simulink model "FYP"  (R2023b)
settings: Solver=FixedStepAuto  StartTime=0.0  StopTime=Inf  RelTol=1e-3  EnableMultiTasking=on
libraries: canmsglib x26, raspberrypiCommlib x26
(part 2 of 4)

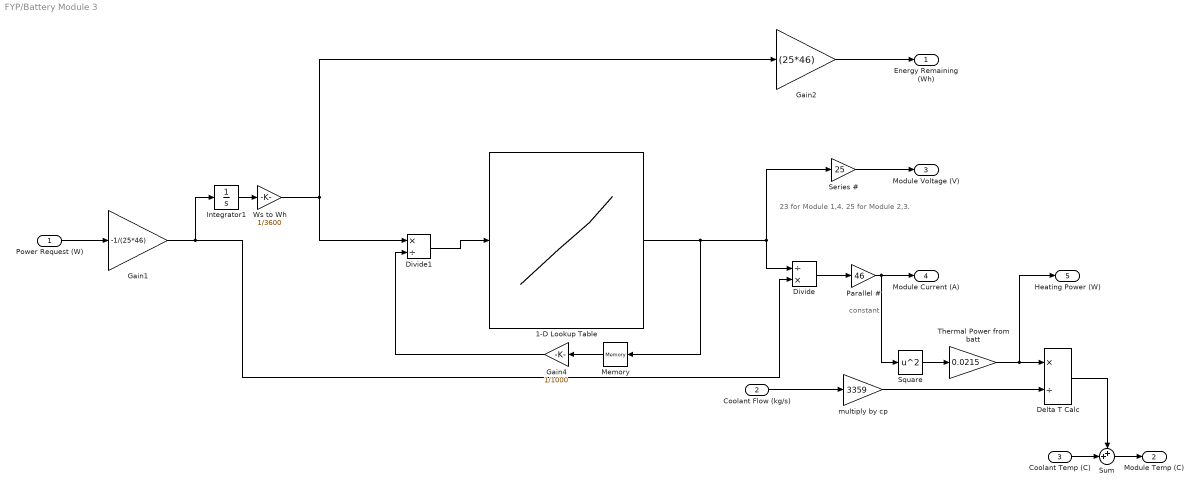
== system FYP/Battery Module 3 ==
  note: constant
  note: 23 for Module 1,4. 25 for Module 2,3.
  Power Request (W) : Inport
  Coolant Flow (kg/s) : Inport  Port=2
  Coolant Temp (C) : Inport  Port=3
  1-D Lookup Table : Lookup_n-D  NumberOfTableDimensions=1  BreakpointsForDimension1=|  Table=|  InternalRulePriority=Speed  RndMeth=Simplest
      BreakpointsForDimension1=|
      | [327.91963
      | 356.24194
      | 389.81097
      | 421.58966
      | 454.48731
      | 486.26599
      | 520.63596
      | 557.87992
      | 595.92482
      | 631.52398
      | 652.73854
      | 690.13124
      | 726.46639
      | 758.34729
      | 795.18499
      | 822.76755
      | 860.65393
      | 891.58806
      | 925.87788
      | 957.35139
      | 996.24173
      | 1029.9537
      | 1071.4861
      | 1113.3355
      | 1155.1849
      | 1197.0343
      | 1238.8837
      |  1280.733
      | 1322.5824
      | 1364.4318
      | 1406.2812
      | 1448.1306
      |   1489.98
      | 1531.8294
      | 1573.6788
      | 1615.5282
      | 1657.3776
      |  1699.227
      | 1741.0764
      | 1782.9257
      | 1824.7751
      | 1866.6245
      | 1908.4739
      | 1950.3233
      | 1992.1727
      | 2034.0221
      | 2075.8715
      | 2117.7209
      | 2174.7882
      | 2212.8331
      | 2254.6825
      | 2296.5319
      | 2338.3813
      | 2380.2307
      | 2422.0801
      | 2463.9295
      | 2505.7789
      | 2547.6283
      | 2589.4777
      |  2631.327
      | 2673.1764
      | 2715.0258
      | 2756.8752
      | 2798.7246
      |  2840.574
      | 2882.4234
      | 2924.2728
      | 2966.1222
      | 3007.9716
      |  3049.821
      | 3091.6704
      | 3133.5197
      | 3175.3691
      | 3217.2185
      | 3259.0679
      | 3300.9173
      | 3342.7667
      | 3384.6161
      | 3426.4655
      | 3468.3149
      | 3510.1643
      | 3552.0137
      | 3593.8631
      | 3635.7124
      | 3677.5618
      | 3719.4112
      | 3761.2606
      |   3803.11
      | 3844.9594
      | 3886.8088
      | 3928.6582
      | 3970.5076
      |  4012.357
      | 4054.2064
      | 4096.0558
      | 4137.9051
      | 4179.7545
      | 4221.6039
      | 4263.4533
      | 4305.3027
      | 4347.1521
      | 4389.0015
      | 4430.8509
      | 4472.7003
      | 4514.5497
      | 4556.3991
      | 4598.2485
      | 4640.0978
      | 4681.9472
      | 4704.0825
      | 4723.7966
      | 4748.3529
      |  4765.646
      | 4785.5464]
      Table=|
      | [2.7985
      | 2.8174
      | 2.8458
      | 2.8738
      | 2.8997
      | 2.9268
      | 2.9549
      | 2.9821
      |  3.009
      | 3.0311
      | 3.0525
      | 3.0727
      | 3.0956
      | 3.1205
      | 3.1365
      | 3.1586
      | 3.1795
      | 3.2002
      | 3.2177
      | 3.2408
      | 3.2608
      | 3.2799
      | 3.3019
      | 3.3209
      |  3.339
      | 3.3545
      | 3.3694
      | 3.3827
      | 3.3945
      | 3.4061
      | 3.4165
      | 3.4265
      |  3.436
      | 3.4452
      | 3.4545
      | 3.4628
      | 3.4712
      |  3.479
      | 3.4866
      | 3.4941
      | 3.5018
      | 3.5098
      | 3.5177
      | 3.5261
      | 3.5347
      | 3.5428
      | 3.5516
      |  3.558
      | 3.5778
      | 3.5818
      |  3.592
      | 3.6021
      | 3.6124
      | 3.6225
      | 3.6324
      | 3.6423
      | 3.6517
      |  3.661
      | 3.6705
      | 3.6797
      | 3.6889
      | 3.6981
      | 3.7063
      | 3.7141
      | 3.7223
      | 3.7297
      | 3.7373
      | 3.7442
      | 3.7511
      | 3.7579
      | 3.7643
      | 3.7711
      | 3.7777
      | 3.7847
      | 3.7916
      | 3.7991
      | 3.8065
      | 3.8143
      | 3.8224
      | 3.8311
      | 3.8405
      | 3.8501
      |   3.86
      | 3.8705
      | 3.8803
      | 3.8902
      |    3.9
      |  3.909
      | 3.9181
      | 3.9258
      | 3.9329
      | 3.9399
      | 3.9456
      | 3.9511
      | 3.9558
      | 3.9603
      | 3.9646
      | 3.9685
      | 3.9719
      |  3.975
      | 3.9783
      | 3.9817
      |  3.986
      | 3.9895
      | 3.9951
      | 4.0003
      | 4.0067
      | 4.0149
      | 4.0239
      | 4.0482
      | 4.0793
      | 4.1102
      | 4.1378
      | 4.1651]
  Delta T Calc : Product  Inputs=*/
  Divide : Product  Inputs=/*
  Divide1 : Product  Inputs=*/
  Gain1 : Gain  Gain=-1/(25*46)
  Gain2 : Gain  Gain=(25*46)
  Gain4 : Gain  Gain=1/1000
  Integrator1 : Integrator  InitialCondition=19.93*3600
  Memory : Memory  InitialCondition=4.1651
  Parallel # : Gain  Gain=46
  Series # : Gain  Gain=25
  Square : Math  Operator=square
  Sum : Sum  Inputs=++|
  Thermal Power from batt : Gain  Gain=0.0215
  Ws to Wh : Gain  Gain=1/3600
  multiply by cp : Gain  Gain=3359
  Energy Remaining (Wh) : Outport
  Module Temp (C) : Outport  Port=2
  Module Voltage (V) : Outport  Port=3
  Module Current (A) : Outport  Port=4
  Heating Power (W) : Outport  Port=5
  wires:
  Power Request (W)/1 -> Gain1/1
  Divide/1 -> Parallel #/1
  Gain1/1 -> Divide/2, Integrator1/1
  Gain2/1 -> Energy Remaining (Wh)/1
  Series #/1 -> Module Voltage (V)/1
  Parallel #/1 -> Square/1, Module Current (A)/1
  Square/1 -> Thermal Power from batt/1
  multiply by cp/1 -> Delta T Calc/2
  Coolant Flow (kg/s)/1 -> multiply by cp/1
  Sum/1 -> Module Temp (C)/1
  Coolant Temp (C)/1 -> Sum/2
  Delta T Calc/1 -> Sum/1
  Thermal Power from batt/1 -> Heating Power (W)/1, Delta T Calc/1
  Divide1/1 -> 1-D Lookup Table/1
  Gain4/1 -> Divide1/2
  1-D Lookup Table/1 -> Memory/1, Divide/1, Series #/1
  Ws to Wh/1 -> Divide1/1, Gain2/1
  Memory/1 -> Gain4/1
  Integrator1/1 -> Ws to Wh/1

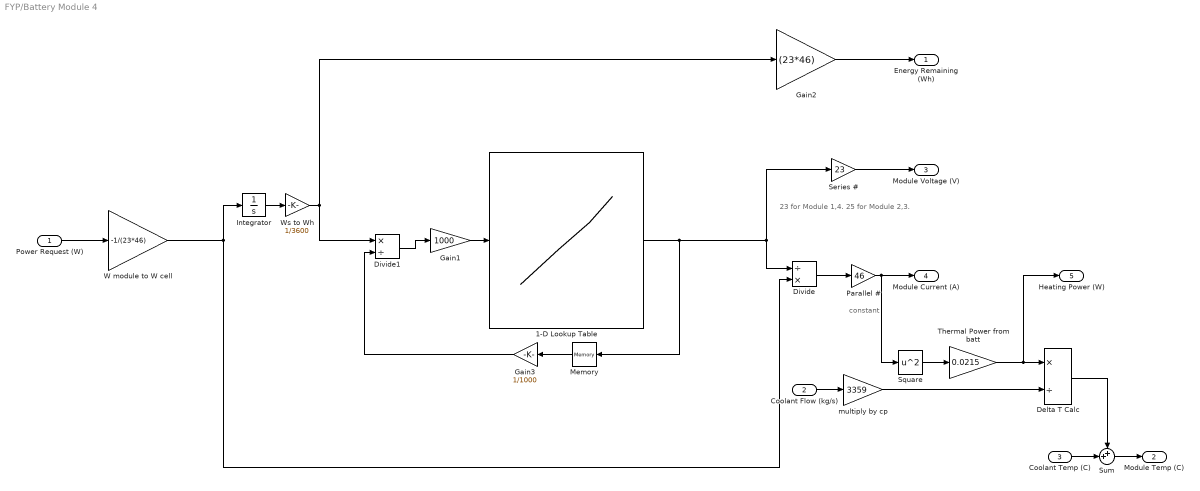
== system FYP/Battery Module 4 ==
  note: constant
  note: 23 for Module 1,4. 25 for Module 2,3.
  Power Request (W) : Inport
  Coolant Flow (kg/s) : Inport  Port=2
  Coolant Temp (C) : Inport  Port=3
  1-D Lookup Table : Lookup_n-D  NumberOfTableDimensions=1  BreakpointsForDimension1=|  Table=|  InternalRulePriority=Speed  RndMeth=Simplest
      BreakpointsForDimension1=|
      | [327.91963
      | 356.24194
      | 389.81097
      | 421.58966
      | 454.48731
      | 486.26599
      | 520.63596
      | 557.87992
      | 595.92482
      | 631.52398
      | 652.73854
      | 690.13124
      | 726.46639
      | 758.34729
      | 795.18499
      | 822.76755
      | 860.65393
      | 891.58806
      | 925.87788
      | 957.35139
      | 996.24173
      | 1029.9537
      | 1071.4861
      | 1113.3355
      | 1155.1849
      | 1197.0343
      | 1238.8837
      |  1280.733
      | 1322.5824
      | 1364.4318
      | 1406.2812
      | 1448.1306
      |   1489.98
      | 1531.8294
      | 1573.6788
      | 1615.5282
      | 1657.3776
      |  1699.227
      | 1741.0764
      | 1782.9257
      | 1824.7751
      | 1866.6245
      | 1908.4739
      | 1950.3233
      | 1992.1727
      | 2034.0221
      | 2075.8715
      | 2117.7209
      | 2174.7882
      | 2212.8331
      | 2254.6825
      | 2296.5319
      | 2338.3813
      | 2380.2307
      | 2422.0801
      | 2463.9295
      | 2505.7789
      | 2547.6283
      | 2589.4777
      |  2631.327
      | 2673.1764
      | 2715.0258
      | 2756.8752
      | 2798.7246
      |  2840.574
      | 2882.4234
      | 2924.2728
      | 2966.1222
      | 3007.9716
      |  3049.821
      | 3091.6704
      | 3133.5197
      | 3175.3691
      | 3217.2185
      | 3259.0679
      | 3300.9173
      | 3342.7667
      | 3384.6161
      | 3426.4655
      | 3468.3149
      | 3510.1643
      | 3552.0137
      | 3593.8631
      | 3635.7124
      | 3677.5618
      | 3719.4112
      | 3761.2606
      |   3803.11
      | 3844.9594
      | 3886.8088
      | 3928.6582
      | 3970.5076
      |  4012.357
      | 4054.2064
      | 4096.0558
      | 4137.9051
      | 4179.7545
      | 4221.6039
      | 4263.4533
      | 4305.3027
      | 4347.1521
      | 4389.0015
      | 4430.8509
      | 4472.7003
      | 4514.5497
      | 4556.3991
      | 4598.2485
      | 4640.0978
      | 4681.9472
      | 4704.0825
      | 4723.7966
      | 4748.3529
      |  4765.646
      | 4785.5464]
      Table=|
      | [2.7985
      | 2.8174
      | 2.8458
      | 2.8738
      | 2.8997
      | 2.9268
      | 2.9549
      | 2.9821
      |  3.009
      | 3.0311
      | 3.0525
      | 3.0727
      | 3.0956
      | 3.1205
      | 3.1365
      | 3.1586
      | 3.1795
      | 3.2002
      | 3.2177
      | 3.2408
      | 3.2608
      | 3.2799
      | 3.3019
      | 3.3209
      |  3.339
      | 3.3545
      | 3.3694
      | 3.3827
      | 3.3945
      | 3.4061
      | 3.4165
      | 3.4265
      |  3.436
      | 3.4452
      | 3.4545
      | 3.4628
      | 3.4712
      |  3.479
      | 3.4866
      | 3.4941
      | 3.5018
      | 3.5098
      | 3.5177
      | 3.5261
      | 3.5347
      | 3.5428
      | 3.5516
      |  3.558
      | 3.5778
      | 3.5818
      |  3.592
      | 3.6021
      | 3.6124
      | 3.6225
      | 3.6324
      | 3.6423
      | 3.6517
      |  3.661
      | 3.6705
      | 3.6797
      | 3.6889
      | 3.6981
      | 3.7063
      | 3.7141
      | 3.7223
      | 3.7297
      | 3.7373
      | 3.7442
      | 3.7511
      | 3.7579
      | 3.7643
      | 3.7711
      | 3.7777
      | 3.7847
      | 3.7916
      | 3.7991
      | 3.8065
      | 3.8143
      | 3.8224
      | 3.8311
      | 3.8405
      | 3.8501
      |   3.86
      | 3.8705
      | 3.8803
      | 3.8902
      |    3.9
      |  3.909
      | 3.9181
      | 3.9258
      | 3.9329
      | 3.9399
      | 3.9456
      | 3.9511
      | 3.9558
      | 3.9603
      | 3.9646
      | 3.9685
      | 3.9719
      |  3.975
      | 3.9783
      | 3.9817
      |  3.986
      | 3.9895
      | 3.9951
      | 4.0003
      | 4.0067
      | 4.0149
      | 4.0239
      | 4.0482
      | 4.0793
      | 4.1102
      | 4.1378
      | 4.1651]
  Delta T Calc : Product  Inputs=*/
  Divide : Product  Inputs=/*
  Divide1 : Product  Inputs=*/
  Gain1 : Gain  Gain=1000
  Gain2 : Gain  Gain=(23*46)
  Gain3 : Gain  Gain=1/1000
  Integrator : Integrator  InitialCondition=19.93*3600
  Memory : Memory  InitialCondition=4.1651
  Parallel # : Gain  Gain=46
  Series # : Gain  Gain=23
  Square : Math  Operator=square
  Sum : Sum  Inputs=++|
  Thermal Power from batt : Gain  Gain=0.0215
  W module to W cell : Gain  Gain=-1/(23*46)
  Ws to Wh : Gain  Gain=1/3600
  multiply by cp : Gain  Gain=3359
  Energy Remaining (Wh) : Outport
  Module Temp (C) : Outport  Port=2
  Module Voltage (V) : Outport  Port=3
  Module Current (A) : Outport  Port=4
  Heating Power (W) : Outport  Port=5
  wires:
  Power Request (W)/1 -> W module to W cell/1
  Divide/1 -> Parallel #/1
  W module to W cell/1 -> Divide/2, Integrator/1
  Gain2/1 -> Energy Remaining (Wh)/1
  Series #/1 -> Module Voltage (V)/1
  Parallel #/1 -> Square/1, Module Current (A)/1
  Square/1 -> Thermal Power from batt/1
  multiply by cp/1 -> Delta T Calc/2
  Coolant Flow (kg/s)/1 -> multiply by cp/1
  Sum/1 -> Module Temp (C)/1
  Coolant Temp (C)/1 -> Sum/2
  Delta T Calc/1 -> Sum/1
  Thermal Power from batt/1 -> Heating Power (W)/1, Delta T Calc/1
  Divide1/1 -> Gain1/1
  Gain3/1 -> Divide1/2
  1-D Lookup Table/1 -> Memory/1, Divide/1, Series #/1
  Ws to Wh/1 -> Divide1/1, Gain2/1
  Memory/1 -> Gain3/1
  Gain1/1 -> 1-D Lookup Table/1
  Integrator/1 -> Ws to Wh/1

== system FYP/Front PT Elec ==
  Battery Voltage : Inport
  Motor Power : Inport  Port=2
  Trigger : TriggerPort  VariantControl=(inherit)
  CAN Pack10 : canmsglib/CAN Pack  CANdbFile=C:\Users\aaron\OneDrive - Loughborough University\Work\Part D\FYP\Model3CAN.dbc  MsgList=ID1A5FrontHVStatus  MsgName=ID1A5FrontHVStatus  MsgIDType=Standard (11-bit identifier)  MsgIdentifier=421  MsgLength=7  Remote=off  ApplyMinMax=off  BusOutput=on  SignalInfo={'DIF_dcCableCurrentEst','24','16','LE','signed','Standard','0','0.1','0','-3276.8','3276.7';'DIF_switchingFrequency','40','11','LE','unsigned','Standard','0','0.01','0','0','20';'DIF_targetFluxMode','51','2','LE','unsigned','Standard','0','1','0','-Inf','Inf';'DIF_vBatQF','10','1','LE','unsigned','Standard','0','1','0','-Inf','Inf';'FrontHighVoltage1A5','0','10','LE','unsigned','Standard','0','0.5','0','0','500';'FrontMotorCurrent1A5','11','11','LE','unsigned','Standard','0','1','0','0','2047'}
      settings: LibrarySourceBlock=canlib/CAN Pack  DataFormat=CANdb specified signals
  CAN Transmit10 : raspberrypiCommlib/CAN Transmit  DeviceID=can0  SetupCAN=off  TypeofCAN=Real  InputDataType=CAN Msg  BlockingMode_=off  BlockTimeout_=1  OutputStatus=off  IdentifierType=Standard (11-bit identifier)  MessageId=100  MsgLength=8  RemoteFrame=off  SimulateUsing=Code generation
  Constant : Constant  Value=0
  Constant1 : Constant  Value=0
  Divide : Product  Inputs=/*
  wires:
  CAN Pack10/1 -> CAN Transmit10/1
  Motor Power/1 -> Divide/2
  Battery Voltage/1 -> CAN Pack10/5, Divide/1
  Divide/1 -> CAN Pack10/6, CAN Pack10/1
  Constant/1 -> CAN Pack10/3
  Constant1/1 -> CAN Pack10/4

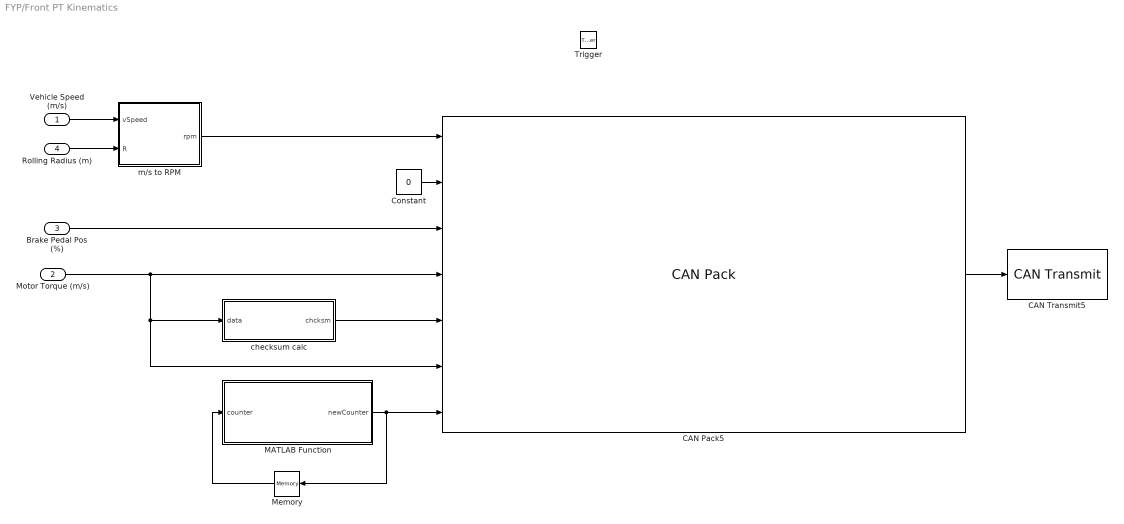
== system FYP/Front PT Kinematics ==
  Vehicle Speed (m/s) : Inport
  Motor Torque (m/s) : Inport  Port=2
  Brake Pedal Pos (%) : Inport  Port=3
  Rolling Radius (m) : Inport  Port=4
  Trigger : TriggerPort  VariantControl=(inherit)
  CAN Pack5 : canmsglib/CAN Pack  CANdbFile=C:\Users\aaron\OneDrive - Loughborough University\Work\Part D\FYP\Model3CAN.dbc  MsgList=ID186DIF_torque  MsgName=ID186DIF_torque  MsgIDType=Standard (11-bit identifier)  MsgIdentifier=390  MsgLength=8  Remote=off  ApplyMinMax=off  BusOutput=on  SignalInfo={'DIF_axleSpeed','40','16','LE','signed','Standard','0','0.1','0','-2750','2750';'DIF_axleSpeedQF','25','1','LE','unsigned','Standard','0','1','0','0','1';'DIF_slavePedalPos','56','8','LE','unsigned','Standard','0','0.4','0','0','100';'DIF_torqueActual','27','13','LE','signed','Standard','0','2','0','-7500','7500';'DIF_torqueChecksum','0','8','LE','unsigned','Standard','0','1','0','0','255';'DIF_torqueCommand','12','13','LE','signed','Standard','0','2','0','-7500','7500';'DIF_torqueCounter','8','4','LE','unsigned','Standard','0','1','0','0','15'}
      settings: LibrarySourceBlock=canlib/CAN Pack  DataFormat=CANdb specified signals
  CAN Transmit5 : raspberrypiCommlib/CAN Transmit  DeviceID=can0  SetupCAN=off  TypeofCAN=Real  InputDataType=CAN Msg  BlockingMode_=off  BlockTimeout_=1  OutputStatus=off  IdentifierType=Standard (11-bit identifier)  MessageId=100  MsgLength=8  RemoteFrame=off  SimulateUsing=Code generation
  Constant : Constant  Value=0
  MATLAB Function : MATLAB Function  TreatAsAtomicUnit=on
  Memory : Memory  InheritSampleTime=on
  checksum calc : MATLAB Function  TreatAsAtomicUnit=on
  m/s to RPM : MATLAB Function  TreatAsAtomicUnit=on
  wires:
  CAN Pack5/1 -> CAN Transmit5/1
  Motor Torque (m/s)/1 -> checksum calc/1(data), CAN Pack5/6, CAN Pack5/4
  Brake Pedal Pos (%)/1 -> CAN Pack5/3
  Constant/1 -> CAN Pack5/2
  Vehicle Speed (m/s)/1 -> m/s to RPM/1(vSpeed)
  m/s to RPM/1(rpm) -> CAN Pack5/1
  Rolling Radius (m)/1 -> m/s to RPM/2(R)
  checksum calc/1(chcksm) -> CAN Pack5/5
  MATLAB Function/1(newCounter) -> Memory/1, CAN Pack5/7
  Memory/1 -> MATLAB Function/1(counter)

== system FYP/Front PT Torque ==
  Motor Torque (Nm) : Inport
  Trigger : TriggerPort  VariantControl=(inherit)
  CAN Pack22 : canmsglib/CAN Pack  CANdbFile=C:\Users\aaron\OneDrive - Loughborough University\Work\Part D\FYP\Model3CAN.dbc  MsgList=ID1D5FrontTorque  MsgName=ID1D5FrontTorque  MsgIDType=Standard (11-bit identifier)  MsgIdentifier=469  MsgLength=8  Remote=off  ApplyMinMax=off  BusOutput=on  SignalInfo={'FrontTorque1D5','21','13','LE','signed','Standard','0','0.222','0','-909.312','909.09';'FrontTorqueRequest1D5','8','13','LE','signed','Standard','0','0.222','0','-909.312','909.09'}
      settings: LibrarySourceBlock=canlib/CAN Pack  DataFormat=CANdb specified signals
  CAN Transmit22 : raspberrypiCommlib/CAN Transmit  DeviceID=can0  SetupCAN=off  TypeofCAN=Real  InputDataType=CAN Msg  BlockingMode_=off  BlockTimeout_=1  OutputStatus=off  IdentifierType=Standard (11-bit identifier)  MessageId=100  MsgLength=8  RemoteFrame=off  SimulateUsing=Code generation
  wires:
  CAN Pack22/1 -> CAN Transmit22/1
  Motor Torque (Nm)/1 -> CAN Pack22/1, CAN Pack22/2

== system FYP/Gear Lever ==
  Gear Lever Pos : Inport
  Trigger : TriggerPort  VariantControl=(inherit)  PortDimensions=1
  CAN Pack37 : canmsglib/CAN Pack  CANdbFile=C:\Users\aaron\OneDrive - Loughborough University\Work\Part D\FYP\tesla sniffing\Model3CAN.dbc  MsgList=ID229GearLever  MsgName=ID229GearLever  MsgIDType=Standard (11-bit identifier)  MsgIdentifier=553  MsgLength=3  Remote=off  ApplyMinMax=off  BusOutput=on  SignalInfo={'GearLeverButton229','16','2','LE','unsigned','Standard','0','1','0','0','3';'GearLeverPosition229','12','3','LE','unsigned','Standard','0','1','0','0','7'}
      settings: LibrarySourceBlock=canlib/CAN Pack  DataFormat=CANdb specified signals
  CAN Transmit37 : raspberrypiCommlib/CAN Transmit  DeviceID=can0  SetupCAN=off  TypeofCAN=Real  InputDataType=CAN Msg  BlockingMode_=off  BlockTimeout_=1  OutputStatus=off  IdentifierType=Standard (11-bit identifier)  MessageId=100  MsgLength=8  RemoteFrame=off  SimulateUsing=Code generation
  Constant : Constant  Value=0
  wires:
  CAN Pack37/1 -> CAN Transmit37/1
  Gear Lever Pos/1 -> CAN Pack37/2
  Constant/1 -> CAN Pack37/1

== system FYP/Range Estimations ==
  SOC : Inport
  Energy : Inport  Port=2
  Trigger : TriggerPort  VariantControl=(inherit)
  CAN Pack90 : canmsglib/CAN Pack  CANdbFile=C:\Users\aaron\OneDrive - Loughborough University\Work\Part D\FYP\tesla sniffing\Model3CAN.dbc  MsgList=ID33AUI_rangeSOC  MsgName=ID33AUI_rangeSOC  MsgIDType=Standard (11-bit identifier)  MsgIdentifier=826  MsgLength=8  Remote=off  ApplyMinMax=off  BusOutput=on  SignalInfo={'UI_Range','0','10','LE','unsigned','Standard','0','1','0','0','1023';'UI_SOC','48','7','LE','unsigned','Standard','0','1','0','0','127';'UI_idealRange','16','10','LE','unsigned','Standard','0','1','0','0','1023';'UI_ratedWHpM','32','10','LE','unsigned','Standard','0','1','0','0','1023';'UI_uSOE','56','7','LE','unsigned','Standard','0','1','0','0','127'}
      settings: LibrarySourceBlock=canlib/CAN Pack  DataFormat=CANdb specified signals
  CAN Transmit90 : raspberrypiCommlib/CAN Transmit  DeviceID=can0  SetupCAN=off  TypeofCAN=Real  InputDataType=CAN Msg  BlockingMode_=off  BlockTimeout_=1  OutputStatus=off  IdentifierType=Standard (11-bit identifier)  MessageId=100  MsgLength=8  RemoteFrame=off  SimulateUsing=Code generation
  MATLAB Function : MATLAB Function  TreatAsAtomicUnit=on
  wires:
  CAN Pack90/1 -> CAN Transmit90/1
  MATLAB Function/1(Range) -> CAN Pack90/1
  MATLAB Function/2(SOC) -> CAN Pack90/2
  MATLAB Function/3(idealRange) -> CAN Pack90/3
  MATLAB Function/4(WHpM) -> CAN Pack90/4
  MATLAB Function/5(uSOE) -> CAN Pack90/5
  SOC/1 -> MATLAB Function/1("SOC ")
  Energy/1 -> MATLAB Function/2(Energy)

== system FYP/Rear PT Elec ==
  Battery Voltage : Inport
  Motor Power : Inport  Port=2
  Trigger : TriggerPort  VariantControl=(inherit)
  CAN Pack10 : canmsglib/CAN Pack  CANdbFile=C:\Users\aaron\OneDrive - Loughborough University\Work\Part D\FYP\tesla sniffing\Model3CAN.dbc  MsgList=ID126RearHVStatus  MsgName=ID126RearHVStatus  MsgIDType=Standard (11-bit identifier)  MsgIdentifier=294  MsgLength=7  Remote=off  ApplyMinMax=off  BusOutput=on  SignalInfo={'DIR_dcCableCurrentEst','24','16','LE','signed','Standard','0','0.1','0','-3276.8','3276.7';'DIR_switchingFrequency','40','11','LE','unsigned','Standard','0','0.01','0','0','20';'DIR_targetFluxMode','51','2','LE','unsigned','Standard','0','1','0','-Inf','Inf';'DIR_vBatQF','10','1','LE','unsigned','Standard','0','1','0','0','1';'RearHighVoltage126','0','10','LE','unsigned','Standard','0','0.5','0','0','500';'RearMotorCurrent126','11','11','LE','unsigned','Standard','0','1','0','0','2047'}
      settings: LibrarySourceBlock=canlib/CAN Pack  DataFormat=CANdb specified signals
  CAN Transmit10 : raspberrypiCommlib/CAN Transmit  DeviceID=can0  SetupCAN=off  TypeofCAN=Real  InputDataType=CAN Msg  BlockingMode_=off  BlockTimeout_=1  OutputStatus=off  IdentifierType=Standard (11-bit identifier)  MessageId=100  MsgLength=8  RemoteFrame=off  SimulateUsing=Code generation
  Constant : Constant  Value=0
  Constant1 : Constant  Value=0
  Divide : Product  Inputs=/*
  wires:
  CAN Pack10/1 -> CAN Transmit10/1
  Motor Power/1 -> Divide/2
  Battery Voltage/1 -> CAN Pack10/5, Divide/1
  Divide/1 -> CAN Pack10/6, CAN Pack10/1
  Constant/1 -> CAN Pack10/3
  Constant1/1 -> CAN Pack10/4

== system FYP/Rear PT Kinematics ==
  Vehicle Speed (m/s) : Inport
  Motor Torque (m/s) : Inport  Port=2
  Brake Pedal Pos (%) : Inport  Port=3
  Rolling Radius (m) : Inport  Port=4
  Trigger : TriggerPort  VariantControl=(inherit)
  CAN Pack5 : canmsglib/CAN Pack  CANdbFile=C:\Users\aaron\OneDrive - Loughborough University\Work\Part D\FYP\tesla sniffing\Model3CAN.dbc  MsgList=ID108DIR_torque  MsgName=ID108DIR_torque  MsgIDType=Standard (11-bit identifier)  MsgIdentifier=264  MsgLength=8  Remote=off  ApplyMinMax=off  BusOutput=on  SignalInfo={'DIR_axleSpeed','40','16','LE','signed','Standard','0','0.1','0','-2750','2750';'DIR_axleSpeedQF','25','1','LE','unsigned','Standard','0','1','0','0','1';'DIR_slavePedalPos','56','8','LE','unsigned','Standard','0','0.4','0','0','100';'DIR_torqueActual','27','13','LE','signed','Standard','0','2','0','-7500','7500';'DIR_torqueChecksum','0','8','LE','unsigned','Standard','0','1','0','0','255';'DIR_torqueCommand','12','13','LE','signed','Standard','0','2','0','-7500','7500';'DIR_torqueCounter','8','4','LE','unsigned','Standard','0','1','0','0','15'}
      settings: LibrarySourceBlock=canlib/CAN Pack  DataFormat=CANdb specified signals
  CAN Transmit5 : raspberrypiCommlib/CAN Transmit  DeviceID=can0  SetupCAN=off  TypeofCAN=Real  InputDataType=CAN Msg  BlockingMode_=off  BlockTimeout_=1  OutputStatus=off  IdentifierType=Standard (11-bit identifier)  MessageId=100  MsgLength=8  RemoteFrame=off  SimulateUsing=Code generation
  Constant : Constant  Value=0
  MATLAB Function : MATLAB Function  TreatAsAtomicUnit=on
  Memory : Memory  InitialCondition=1  InheritSampleTime=on
  checksum calc : MATLAB Function  TreatAsAtomicUnit=on
  m/s to RPM : MATLAB Function  TreatAsAtomicUnit=on
  wires:
  CAN Pack5/1 -> CAN Transmit5/1
  Motor Torque (m/s)/1 -> checksum calc/1(data), CAN Pack5/6, CAN Pack5/4
  Brake Pedal Pos (%)/1 -> CAN Pack5/3
  Constant/1 -> CAN Pack5/2
  Vehicle Speed (m/s)/1 -> m/s to RPM/1(vSpeed)
  m/s to RPM/1(rpm) -> CAN Pack5/1
  Rolling Radius (m)/1 -> m/s to RPM/2(R)
  checksum calc/1(chcksm) -> CAN Pack5/5
  MATLAB Function/1(newCounter) -> Memory/1, CAN Pack5/7
  Memory/1 -> MATLAB Function/1(counter)

== system FYP/Rear PT Torque ==
  Motor Torque (Nm) : Inport
  Trigger : TriggerPort  VariantControl=(inherit)
  CAN Pack22 : canmsglib/CAN Pack  CANdbFile=C:\Users\aaron\OneDrive - Loughborough University\Work\Part D\FYP\tesla sniffing\Model3CAN.dbc  MsgList=ID1D8RearTorque  MsgName=ID1D8RearTorque  MsgIDType=Standard (11-bit identifier)  MsgIdentifier=472  MsgLength=8  Remote=off  ApplyMinMax=off  BusOutput=on  SignalInfo={'Checksum1D8','56','8','LE','unsigned','Standard','0','1','0','0','255';'Counter1D8','53','3','LE','unsigned','Standard','0','1','0','0','7';'RearTorque1D8','21','13','LE','signed','Standard','0','0.222','0','-909.312','909.09';'RearTorqueRequest1D8','8','13','LE','signed','Standard','0','0.222','0','-909.312','909.09';'TorqueFlags1D8','0','8','LE','unsigned','Standard','0','1','0','0','255'}
      settings: LibrarySourceBlock=canlib/CAN Pack  DataFormat=CANdb specified signals
  CAN Transmit22 : raspberrypiCommlib/CAN Transmit  DeviceID=can0  SetupCAN=off  TypeofCAN=Real  InputDataType=CAN Msg  BlockingMode_=off  BlockTimeout_=1  OutputStatus=off  IdentifierType=Standard (11-bit identifier)  MessageId=100  MsgLength=8  RemoteFrame=off  SimulateUsing=Code generation
  Constant : Constant  Value=0
  MATLAB Function : MATLAB Function  TreatAsAtomicUnit=on
  Memory : Memory  InheritSampleTime=on
  checksum calc : MATLAB Function  TreatAsAtomicUnit=on
  wires:
  CAN Pack22/1 -> CAN Transmit22/1
  Motor Torque (Nm)/1 -> CAN Pack22/3, CAN Pack22/4, checksum calc/1(data)
  checksum calc/1(chcksm) -> CAN Pack22/1
  Memory/1 -> MATLAB Function/1(counter)
  MATLAB Function/1(newCounter) -> Memory/1, CAN Pack22/2
  Constant/1 -> CAN Pack22/5

== system FYP/Subsystem ==
  vehicle displacement (m) : Inport
  Trigger : TriggerPort  VariantControl=(inherit)  PortDimensions=1
  CAN Pack102 : canmsglib/CAN Pack  CANdbFile=C:\Users\aaron\OneDrive - Loughborough University\Work\Part D\FYP\tesla sniffing\Model3CAN.dbc  MsgList=ID3B6odometer  MsgName=ID3B6odometer  MsgIDType=Standard (11-bit identifier)  MsgIdentifier=950  MsgLength=4  Remote=off  ApplyMinMax=off  BusOutput=on  SignalInfo={'Odometer3B6','0','32','LE','unsigned','Standard','0','0.001','0','0','4294970'}
      settings: LibrarySourceBlock=canlib/CAN Pack  DataFormat=CANdb specified signals
  CAN Transmit102 : raspberrypiCommlib/CAN Transmit  DeviceID=can0  SetupCAN=off  TypeofCAN=Real  InputDataType=CAN Msg  BlockingMode_=off  BlockTimeout_=1  OutputStatus=off  IdentifierType=Standard (11-bit identifier)  MessageId=100  MsgLength=8  RemoteFrame=off  SimulateUsing=Code generation
  Gain : Gain  Gain=1/1000
  wires:
  CAN Pack102/1 -> CAN Transmit102/1
  vehicle displacement (m)/1 -> Gain/1
  Gain/1 -> CAN Pack102/1

== system FYP/Subsystem1 ==
  vehicle speed : Inport
  Trigger : TriggerPort  VariantControl=(inherit)  PortDimensions=1
  CAN Pack48 : canmsglib/CAN Pack  CANdbFile=C:\Users\aaron\OneDrive - Loughborough University\Work\Part D\FYP\tesla sniffing\Model3CAN.dbc  MsgList=ID257DIspeed  MsgName=ID257DIspeed  MsgIDType=Standard (11-bit identifier)  MsgIdentifier=599  MsgLength=8  Remote=off  ApplyMinMax=off  BusOutput=on  SignalInfo={'DI_speedChecksum','0','8','LE','unsigned','Standard','0','1','0','0','255';'DI_speedCounter','8','4','LE','unsigned','Standard','0','1','0','0','15';'DI_uiSpeed','24','9','LE','unsigned','Standard','0','1','0','0','510';'DI_uiSpeedHighSpeed','34','9','LE','unsigned','Standard','0','1','0','0','510';'DI_uiSpeedUnits','33','1','LE','unsigned','Standard','0','1','0','0','1';'DI_vehicleSpeed','12','12','LE','unsigned','Standard','0','0.08','-40','-40','285'}
      settings: LibrarySourceBlock=canlib/CAN Pack  DataFormat=CANdb specified signals
  CAN Transmit48 : raspberrypiCommlib/CAN Transmit  DeviceID=can0  SetupCAN=off  TypeofCAN=Real  InputDataType=CAN Msg  BlockingMode_=off  BlockTimeout_=1  OutputStatus=off  IdentifierType=Standard (11-bit identifier)  MessageId=100  MsgLength=8  RemoteFrame=off  SimulateUsing=Code generation
  Constant : Constant
  MATLAB Function : MATLAB Function  TreatAsAtomicUnit=on
  MATLAB Function1 : MATLAB Function  TreatAsAtomicUnit=on
  Memory : Memory  InitialCondition=1  InheritSampleTime=on
  checksum calc : MATLAB Function  TreatAsAtomicUnit=on
  wires:
  CAN Pack48/1 -> CAN Transmit48/1
  vehicle speed/1 -> MATLAB Function1/1(v), checksum calc/1(data), CAN Pack48/6
  Constant/1 -> CAN Pack48/5
  MATLAB Function/1(newCounter) -> CAN Pack48/2, Memory/1
  checksum calc/1(chcksm) -> CAN Pack48/1
  Memory/1 -> MATLAB Function/1(counter)
  MATLAB Function1/2(hsSpeed) -> CAN Pack48/4
  MATLAB Function1/1(Speed) -> CAN Pack48/3

== system FYP/Vehicle Estimates ==
  Vehicle Mass : Inport
  Trigger : TriggerPort  VariantControl=(inherit)
  CAN Pack53 : canmsglib/CAN Pack  CANdbFile=C:\Users\aaron\OneDrive - Loughborough University\Work\Part D\FYP\tesla sniffing\Model3CAN.dbc  MsgList=ID267DI_vehicleEstimates  MsgName=ID267DI_vehicleEstimates  MsgIDType=Standard (11-bit identifier)  MsgIdentifier=615  MsgLength=8  Remote=off  ApplyMinMax=off  BusOutput=on  SignalInfo={'DI_gradeEst','33','7','LE','signed','Standard','0','1','0','-40','40';'DI_gradeEstInternal','48','7','LE','signed','Standard','0','1','0','-40','40';'DI_mass','0','10','LE','unsigned','Standard','0','5','1900','1900','7010';'DI_massConfidence','32','1','LE','unsigned','Standard','0','1','0','0','1';'DI_relativeTireTreadDepth','16','6','LE','signed','Standard','0','0.2','0','-6.2','6.2';'DI_steeringAngleOffset','56','8','LE','signed','Standard','0','0.2','0','-25.6','25.4';'DI_tireFitment','10','2','LE','unsigned','Standard','0','1','0','0','3';'DI_trailerDetected','12','1','LE','unsigned','Standard','0','1','0','0','1';'DI_vehicleEstimatesChecksum','40','8','LE','unsigned','Standard','0','1','0','0','255';'DI_vehicleEstimatesCounter','13','3','LE','unsigned','Standard','0','1','0','0','7'}
      settings: LibrarySourceBlock=canlib/CAN Pack  DataFormat=CANdb specified signals
  CAN Transmit53 : raspberrypiCommlib/CAN Transmit  DeviceID=can0  SetupCAN=off  TypeofCAN=Real  InputDataType=CAN Msg  BlockingMode_=off  BlockTimeout_=1  OutputStatus=off  IdentifierType=Standard (11-bit identifier)  MessageId=100  MsgLength=8  RemoteFrame=off  SimulateUsing=Code generation
  Constant : Constant  Value=0
  Digital Clock : DigitalClock  SampleTime=-1
  MATLAB Function : MATLAB Function  TreatAsAtomicUnit=on
  Memory : Memory  InitialCondition=1  InheritSampleTime=on
  checksum calc : MATLAB Function  TreatAsAtomicUnit=on
  wires:
  CAN Pack53/1 -> CAN Transmit53/1
  Constant/1 -> CAN Pack53/4, CAN Pack53/5, CAN Pack53/7, CAN Pack53/8, CAN Pack53/6, CAN Pack53/2, CAN Pack53/1
  Vehicle Mass/1 -> CAN Pack53/3
  Memory/1 -> MATLAB Function/1(counter)
  MATLAB Function/1(newCounter) -> CAN Pack53/10, Memory/1
  checksum calc/1(chcksm) -> CAN Pack53/9
  Digital Clock/1 -> checksum calc/1(data)
